simulink model "prueba_para_th"  (R2018a)
settings: Solver=VariableStepAuto  StartTime=0.0  StopTime=0.5  RelTol=1e-3
settings Model: Creator=cmparedes  LastModifiedBy=cmparedes

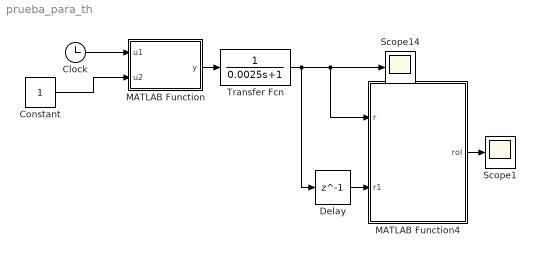
== system prueba_para_th ==
  Clock : Clock
  Constant : Constant
  Delay : Delay  DelayLength=1
  MATLAB Function : MATLAB Function  TreatAsAtomicUnit=on
  MATLAB Function4 : MATLAB Function  TreatAsAtomicUnit=on
  Scope1 : Scope
  Scope14 : Scope
  Transfer Fcn : TransferFcn  Denominator=[0.0025 1]
  wires:
  Clock/1 -> MATLAB Function/1(u1)
  Constant/1 -> MATLAB Function/2(u2)
  MATLAB Function/1(y) -> Transfer Fcn/1
  Transfer Fcn/1 -> Delay/1, MATLAB Function4/1(r), Scope14/1
  MATLAB Function4/1(rol) -> Scope1/1
  Delay/1 -> MATLAB Function4/2(r1)

== matlab function prueba_para_th/MATLAB Function4 ==
  data: r input; rol output; r1 input
function rol = fcn(r,r1)%u1,u2,ym1,ym2)
Th_det = 6.5e-8;
m=r-r1;
if m>0
    Th_det=0.01;  %2.5
elseif m<0  && r<=0.7
    Th_det=0.9; 
end


% sys=tf(1,[0.001 1]);


if r >=Th_det
    rol=1;
else
    rol=0;
end

== matlab function prueba_para_th/MATLAB Function ==
  data: u1 input; y output; u2 input
function y = fcn(u1,u2)
if u1>=0.10 && u1<=0.2%u1>=1000
    y=1;
else
    y = 0;

end
